simulink model "Q8_Model_2015a"  (R2015a)
settings: Solver=ode45  SolverMode=SingleTasking  StartTime=0.0  StopTime=10.0  RelTol=1e-3
values from neighbouring files (symbols this model uses):
  D = [0 0]'    [main.m]
  K = lqr(A_aug, B_aug, Qr, Rr)    [main_sim.m]
  L = lqe(A, G, C, Qe, Re)    [main.m]    (also in main_sim.m)
  x0 = [0.1 0 0 0 0]'    [main.m]    (also in main_sim.m = [alpha_init 0 beta_init 0 0])
undefined symbols (not defined in the file or in its folder): A, B, C
settings Model: CovMetricSettings=dwe  CovHtmlReporting=off  covSaveCumulativeToWorkspaceVar=off  CovSaveSingleToWorkspaceVar=off  CovExternalEMLEnable=on  Creator=lucas  LastModifiedBy=Tomas Teixeira
settings DataIOCC: LimitDataPoints=off  SaveFormat=Dataset  ReturnWorkspaceOutputs=on
settings DebuggingCC: UnconnectedInputMsg=none  UnconnectedOutputMsg=none  UnconnectedLineMsg=none  SFUnexpectedBacktrackingDiag=error  SFNoUnconditionalDefaultTransitionDiag=error
settings HardwareCC: ProdBitPerPointer=64  ProdLargestAtomicFloat=Float  ProdIntDivRoundTo=Zero  ProdEndianess=LittleEndian  ProdHWDeviceType=Specified
settings ModelReferenceCC: PropagateSignalLabelsOutOfModel=on
settings SFSimCC: SimUseLocalCustomCode=on
settings RTWCC: RTWUseLocalCustomCode=on
settings GRTTargetCC: TargetLangStandard=C99 (ISO)

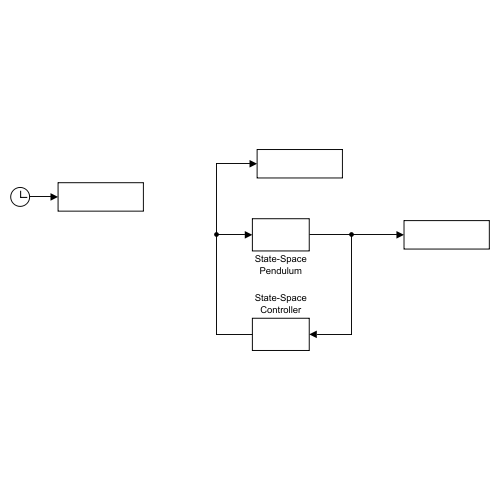
[thumbnail: Simulink's stored preview of the top-level diagram]
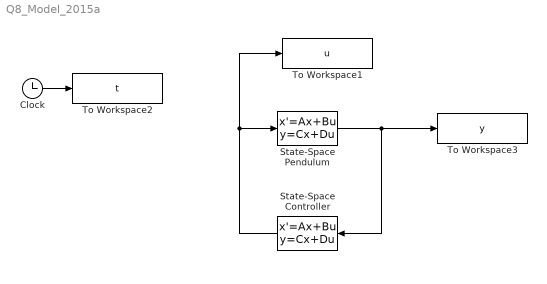
== system Q8_Model_2015a ==
  Clock : Clock
  State-Space Controller : StateSpace  A=A - B*K - L*C  B=L  C=-K  D=[0 0]  X0=0  ContinuousStateAttributes={'y1','y2','y3','y4','y5'}
  State-Space Pendulum : StateSpace  A=A  B=B  C=C  D=D  X0=x0  ContinuousStateAttributes={'x1','x2','x3','x4','x5'}
  To Workspace1 : ToWorkspace  VariableName=u  SaveFormat=Timeseries  SampleTime=-1
  To Workspace2 : ToWorkspace  VariableName=t  SaveFormat=Timeseries  SampleTime=-1
  To Workspace3 : ToWorkspace  VariableName=y  SaveFormat=Timeseries  SampleTime=-1
  wires:
  State-Space Pendulum/1 -> To Workspace3/1, State-Space Controller/1
  State-Space Controller/1 -> To Workspace1/1, State-Space Pendulum/1
  Clock/1 -> To Workspace2/1
